simulink model "Hardware_Hidden_Symulink"  (R2022a)
settings: Solver=FixedStepAuto  StartTime=0.0  StopTime=10  FixedStep=1e-3  RelTol=1e-3  EnableMultiTasking=on
undefined symbols (not defined in the file): a, A0, A1, b, c, D0, D1, D10, D11, D12, D13, D2, D3, D5, D6, D8, D9, PTA0, PTA1, PTA2, PTB2, PTB3, PTB9, PTC16, PTC17, PTC2, PTC4, PTD0, PTD1, PTD2, PTD3
libraries: frdmk64flib x19, simulink x1, hdlsllib x1
settings Model: ExtModeTrigDuration=5  Creator=pauls  LastModifiedBy=eddys
settings OptimizationCC: EnhancedBackFolding=on  PassReuseOutputArgsAs=Individual arguments  ZeroExternalMemoryAtStartup=off  ZeroInternalMemoryAtStartup=off  MaxStackSize=64  OptimizeBlockOrder=speed  DifferentSizesBufferReuse=on  OptimizationCustomize=off  EfficientTunableParamExpr=on
settings DebuggingCC: ParameterTunabilityLossMsg=error  UnderSpecifiedDimensionMsg=warning
settings HardwareCC: ProdBitPerPointer=32  ProdBitPerSizeT=32  ProdBitPerPtrDiffT=32  ProdLargestAtomicInteger=Long  ProdLargestAtomicFloat=Double  ProdWordSize=32  ProdHWDeviceType=ARM Compatible->ARM Cortex
settings SFSimCC: MATLABDynamicMemAlloc=off
settings RTWCC: SystemTargetFile=ert.tlc  HardwareBoard=NXP FRDM-K64F  TLCOptions="-aInlineSetEventsForThisBaseRateFcn=TLC_FALSE -aSuppressMultiTaskScheduler=TLC_FALSE  -aRateBasedStepFcn=0"  TemplateMakefile=ert_default_tmf  Toolchain=GNU Tools for ARM Embedded Processors
settings CodeAppCC: ForceParamTrailComments=on  IgnoreCustomStorageClasses=off  OperatorAnnotations=on  SimulinkDataObjDesc=on  SFDataObjDesc=on  InsertBlockDesc=on
settings ERTTargetCC: ExtModeTransport=4  ExtModeMexFile=sendToCommService

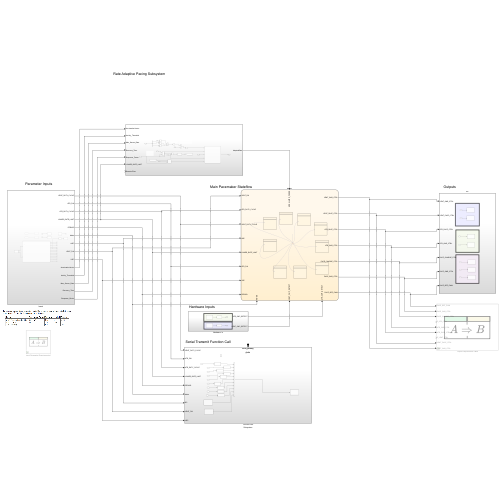
[thumbnail: Simulink's stored preview of the top-level diagram]
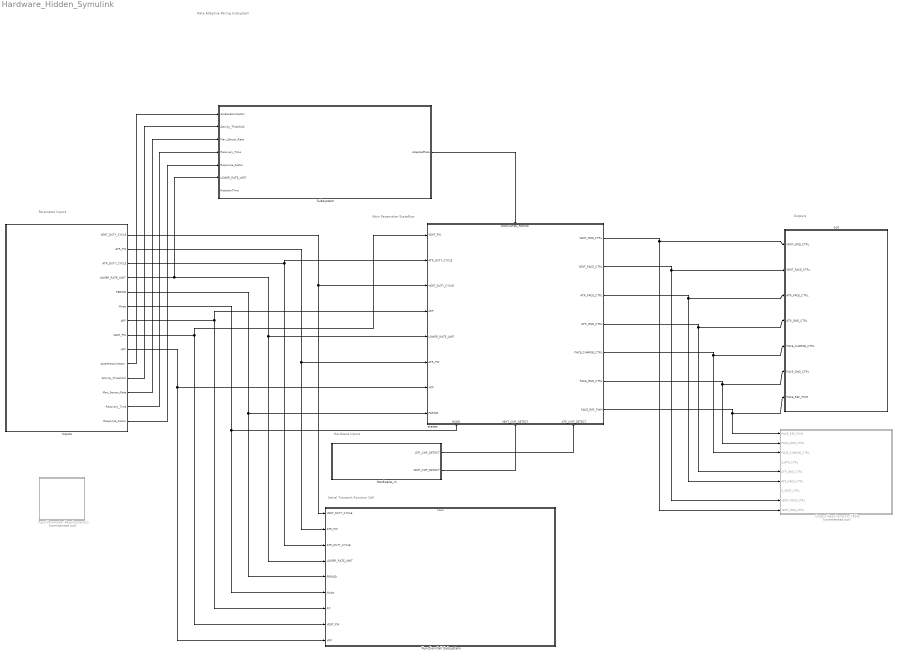
== system Hardware_Hidden_Symulink ==
  note: Rate Adaptive Pacing Subsystem
  note: Serial Transmit Function Call
  note: Main Pacemaker Stateflow
  note: Outputs
  note: Hardware Inputs
  note: Parameter Inputs
  " states  " : Stateflow chart  TreatAsAtomicUnit=on
      settings: PortSchema="{\"entries\":[{\"content\":{\"sides\":[{\"content\":{\"connectorIds\":[\"In4\",\"In6\",\"In5\",\"In10\",\"In11\",\"In7\",\"In9\",\"In8\"]},\"type\":\"ConnectorPlacement.EquallySpacedRectSide\",\"uuid\":\"01118a3a-35ab-415d-a4dc-7a9e5022dc58\"},{\"content\":{\"connectorIds\":[\"Out1\",\"Out2\",\"Out3\",\"Out4\",\"Out5\",\"Out6\",\"Out7\"],\"side\":\"RIGHT\"},\"type\":\"ConnectorPlacement.EquallySpacedRectSide\",\"uuid\":\"d119b6db-c579-45b6-8580-2a3960ab3129\"},{\"content\":{\"connectorIds\":[\"In12\"],\"side\":\"TOP\"},\"type\":\"ConnectorPlacement.EquallySpacedRectSide\",\"uuid\":\"18fa5379-1691-4053-811b-8d647a346445\"},{\"content\":{\"connectorIds\":[\"In1\",\"In3\",\"In2\"],\"side\":\"BOTTOM\"},\"type\":\"ConnectorPlacement.EquallySpacedRectSide\",\"uuid\":\"c19ca9f7-b829-4e11-b03e-3e9d42b35795\"}]},\"type\":\"ConnectorPlacement.EquallySpacedConnector\",\"uuid\":\"6e6fa963-33ea-4c14-97b4-73e5587667a9\"}],\"packageUris\":[\"http://schema.mathworks.com/mf0/Connector/R2020b\"],\"version\":\"1.0\"}"
  Function-Call Subsystem : Subsystem  TreatAsAtomicUnit=on
  Hardware_in : Subsystem
  Input Parameter Requirements1 : Requirements Table  Commented=on  TreatAsAtomicUnit=on
  Inputs : Subsystem
  Output Requirements Table : Requirements Table  Commented=on  TreatAsAtomicUnit=on
  Subsystem : Subsystem
  "out " : Subsystem
  wires:
  Inputs/5(PERIOD) -> Function-Call Subsystem/5(PERIOD), " states  "/8(PERIOD)
  Inputs/4(LOWER_RATE_LIMIT) -> Subsystem/6(LOWER_RATE_LIMIT), Function-Call Subsystem/4(LOWER_RATE_LIMIT), " states  "/11(LOWER_RATE_LIMIT)
  Inputs/1(VENT_DUTY_CYCLE) -> Function-Call Subsystem/1(VENT_DUTY_CYCLE), " states  "/5(VENT_DUTY_CYCLE)
  Inputs/7(ARP) -> Function-Call Subsystem/7(RP), " states  "/10(ARP)
  Inputs/3(ATR_DUTY_CYCLE) -> Function-Call Subsystem/3(ATR_DUTY_CYCLE), " states  "/6(ATR_DUTY_CYCLE)
  Hardware_in/2(VENT_CMP_DETECT) -> " states  "/3(VENT_CMP_DETECT)
  Inputs/2(ATR_PW) -> Function-Call Subsystem/2(ATR_PW), " states  "/7(ATR_PW)
  Hardware_in/1(ATR_CMP_DETECT) -> " states  "/2(ATR_CMP_DETECT)
  Inputs/6(Mode) -> Function-Call Subsystem/6(Mode), " states  "/1(MODE)
  Inputs/8(VENT_PW) -> Function-Call Subsystem/8(VENT_PW), " states  "/4(VENT_PW)
  Inputs/9(VRP) -> Function-Call Subsystem/9(VRP), " states  "/9(VRP)
  " states  "/2(VENT_PACE_CTRL) -> "out "/2(VENT_PACE_CTRL), Output Requirements Table/8(VENT_PACE_CTRL)
  " states  "/7(PACE_REF_PWM) -> Output Requirements Table/1(PACE_REF_PWM), "out "/7(PACE_REF_PWM)
  " states  "/1(VENT_GND_CTRL) -> Output Requirements Table/9(VENT_GND_CTRL), "out "/1(VENT_GND_CTRL)
  " states  "/6(PACE_GND_CTRL) -> Output Requirements Table/2(PACE_GND_CTRL), "out "/6(PACE_GND_CTRL)
  " states  "/3(ATR_PACE_CTRL) -> Output Requirements Table/6(ATR_PACE_CTRL), "out "/3(ATR_PACE_CTRL)
  " states  "/4(ATR_GND_CTRL) -> "out "/4(ATR_GND_CTRL), Output Requirements Table/5(ATR_GND_CTRL)
  " states  "/5(PACE_CHARGE_CTRL) -> Output Requirements Table/3(PACE_CHARGE_CTRL), "out "/5(PACE_CHARGE_CTRL)
  Inputs/10(AccelerationVector) -> Subsystem/1(AccelerationVector)
  Inputs/11(Activity_Threshold) -> Subsystem/2(Activity_Threshold)
  Inputs/12(Max_Sensor_Rate) -> Subsystem/3(Max_Sensor_Rate)
  Inputs/13(Recovery_Time) -> Subsystem/4(Recovery_Time)
  Inputs/14(Response_Factor) -> Subsystem/5(Response_Factor)
  Subsystem/1(AdaptedRate) -> " states  "/12(MODULATED_PERIOD)

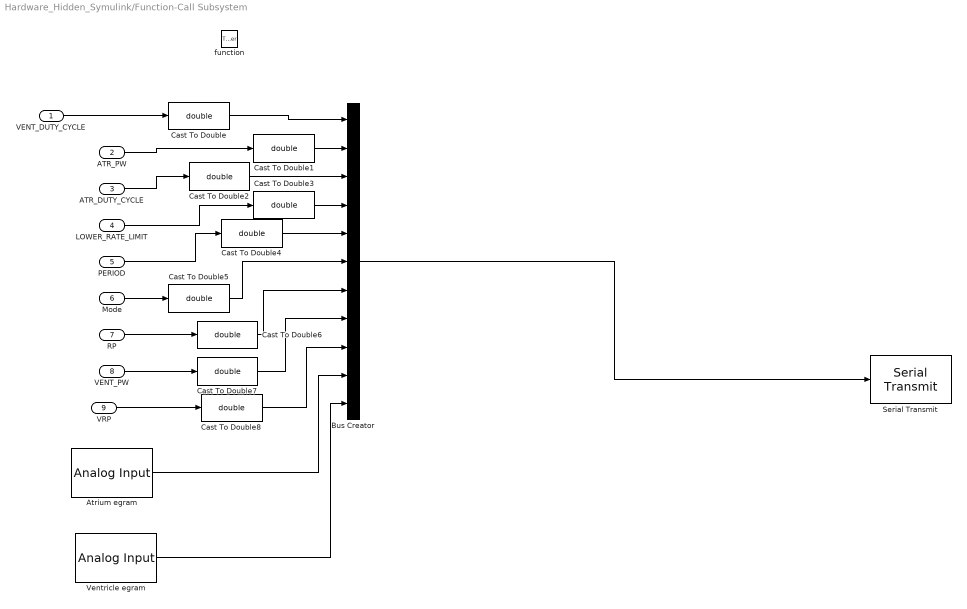
== system Hardware_Hidden_Symulink/Function-Call Subsystem ==
  VENT_DUTY_CYCLE : Inport
  ATR_PW : Inport  Port=2
  ATR_DUTY_CYCLE : Inport  Port=3
  LOWER_RATE_LIMIT : Inport  Port=4
  PERIOD : Inport  Port=5
  Mode : Inport  Port=6
  RP : Inport  Port=7
  VENT_PW : Inport  Port=8
  VRP : Inport  Port=9
  function : TriggerPort  TriggerType=function-call  IsSimulinkFunction=on  FunctionName=send_param  VariantControl=(inherit)
  Atrium egram : frdmk64flib/Analog Input  Whichpin=PTB2 (A0)  SampleTime=-1
  Bus Creator : BusCreator  Inputs=11
  Cast To Double{,1..8} (9 alike) : DataTypeConversion  OutDataTypeStr=double  SaturateOnIntegerOverflow=off  RndMeth=Floor
  Serial Transmit : frdmk64flib/Serial Transmit  SCIModule=0  Baudrate=uint32(9600)  Parity=None  StopBits=1  HardwareFlowControl=None  ByteOrder=LittleEndian  BlockingMode=on  OutputStatus=off
  Ventricle egram : frdmk64flib/Analog Input  Whichpin=PTB3 (A1)  SampleTime=-1
  wires:
  ATR_PW/1 -> Cast To Double1/1
  LOWER_RATE_LIMIT/1 -> Cast To Double3/1
  PERIOD/1 -> Cast To Double4/1
  Mode/1 -> Cast To Double5/1
  RP/1 -> Cast To Double6/1
  VENT_PW/1 -> Cast To Double7/1
  VRP/1 -> Cast To Double8/1
  Bus Creator/1 -> Serial Transmit/1
  Atrium egram/1 -> Bus Creator/10
  Ventricle egram/1 -> Bus Creator/11
  Cast To Double1/1 -> Bus Creator/2
  Cast To Double3/1 -> Bus Creator/4
  Cast To Double4/1 -> Bus Creator/5
  Cast To Double5/1 -> Bus Creator/6
  Cast To Double6/1 -> Bus Creator/7
  Cast To Double7/1 -> Bus Creator/8
  Cast To Double8/1 -> Bus Creator/9
  VENT_DUTY_CYCLE/1 -> Cast To Double/1
  Cast To Double/1 -> Bus Creator/1
  ATR_DUTY_CYCLE/1 -> Cast To Double2/1
  Cast To Double2/1 -> Bus Creator/3

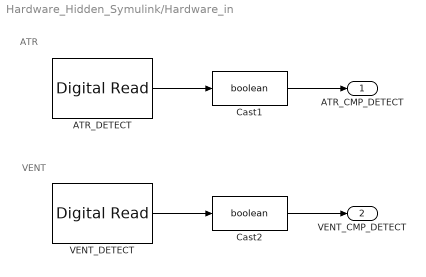
== system Hardware_Hidden_Symulink/Hardware_in ==
  note: VENT
  note: ATR
  ATR_DETECT : frdmk64flib/Digital Read  Whichpin=PTC16 (D0)  SampleTime=-1
  Cast1 : DataTypeConversion  OutDataTypeStr=boolean  SaturateOnIntegerOverflow=off  RndMeth=Floor
  Cast2 : DataTypeConversion  OutDataTypeStr=boolean  SaturateOnIntegerOverflow=off  RndMeth=Floor
  VENT_DETECT : frdmk64flib/Digital Read  Whichpin=PTC17 (D1)  SampleTime=-1
  ATR_CMP_DETECT : Outport
  VENT_CMP_DETECT : Outport  Port=2
  wires:
  Cast1/1 -> ATR_CMP_DETECT/1
  ATR_DETECT/1 -> Cast1/1
  VENT_DETECT/1 -> Cast2/1
  Cast2/1 -> VENT_CMP_DETECT/1

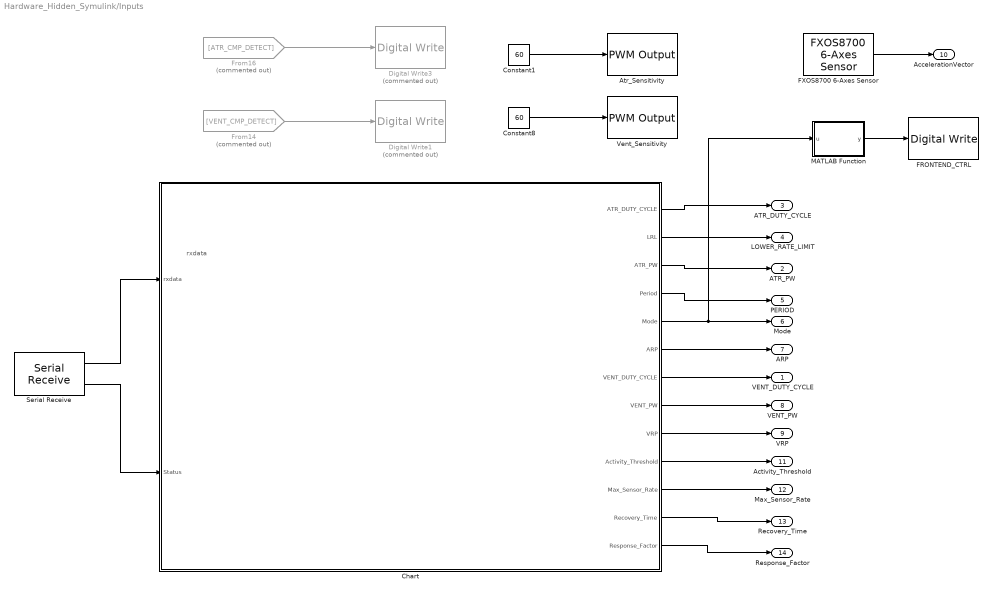
== system Hardware_Hidden_Symulink/Inputs ==
  note: rxdata
  Atr_Sensitivity : frdmk64flib/PWM Output  Whichpin=PTA1 (D3)  InitialFrequency=2000  InitialDutyCycle=0
  Chart : Stateflow chart  TreatAsAtomicUnit=on
      settings: PortSchema="{\"entries\":[{\"content\":{\"sides\":[{\"content\":{\"connectorIds\":[\"In2\",\"In1\"]},\"type\":\"ConnectorPlacement.EquallySpacedRectSide\",\"uuid\":\"d1877822-3205-4f6f-9701-98b371c9c093\"},{\"content\":{\"connectorIds\":[\"Out1\",\"Out2\",\"Out3\",\"Out13\",\"Out4\",\"Out5\",\"Out6\",\"Out7\",\"Out8\",\"Out9\",\"Out10\",\"Out11\",\"Out12\"],\"side\":\"RIGHT\"},\"type\":\"ConnectorPlacement.EquallySpacedRectSide\",\"uuid\":\"d3b9604d-8d2f-41ee-8af9-f72c4df8ba57\"},{\"content\":{\"connectorIds\":[],\"side\":\"TOP\"},\"type\":\"ConnectorPlacement.EquallySpacedRectSide\",\"uuid\":\"4e9204c9-b50b-48f8-942a-bbb1a82b0f42\"}]},\"type\":\"ConnectorPlacement.EquallySpacedConnector\",\"uuid\":\"d64fca82-a3a4-4877-a2ac-6316b03fcfcd\"}],\"packageUris\":[\"http://schema.mathworks.com/mf0/Connector/R2020b\"],\"version\":\"1.0\"}"
  Constant1 : Constant  Value=60
  Constant8 : Constant  Value=60
  Digital Write1 : frdmk64flib/Digital Write  Commented=on  Whichpin=GREEN_LED
  Digital Write3 : frdmk64flib/Digital Write  Commented=on  Whichpin=BLUE_LED
  FRONTEND_CTRL : frdmk64flib/Digital Write  Whichpin=PTD1 (D13)
  FXOS8700 6-Axes Sensor : frdmk64flib/FXOS8700 6-Axes Sensor  Activesensor=Accelerometer only  ODR=800Hz  HybridODR=400Hz  Accelfullrange=-4g to +4g  SampleTime=-1
  From14 : From  Commented=on  GotoTag=VENT_CMP_DETECT
  From16 : From  Commented=on  GotoTag=ATR_CMP_DETECT
  MATLAB Function : MATLAB Function  TreatAsAtomicUnit=on
  Serial Receive : frdmk64flib/Serial Receive  SCIModule=0  Baudrate=uint32(9600)  Parity=None  StopBits=1  HardwareFlowControl=None  ByteOrder=LittleEndian  DataType=uint8  DataLength=19  BlockingMode=off  OutputStatus=on  SampleTime=0.1
  Vent_Sensitivity : frdmk64flib/PWM Output  Whichpin=PTC2 (D6)  InitialFrequency=2000  InitialDutyCycle=0
  VENT_DUTY_CYCLE : Outport
  ATR_PW : Outport  Port=2
  ATR_DUTY_CYCLE : Outport  Port=3
  LOWER_RATE_LIMIT : Outport  Port=4
  PERIOD : Outport  Port=5
  Mode : Outport  Port=6
  ARP : Outport  Port=7
  VENT_PW : Outport  Port=8
  VRP : Outport  Port=9
  AccelerationVector : Outport  Port=10
  Activity_Threshold : Outport  Port=11
  Max_Sensor_Rate : Outport  Port=12
  Recovery_Time : Outport  Port=13
  Response_Factor : Outport  Port=14
  wires:
  From14/1 -> Digital Write1/1
  Constant8/1 -> Vent_Sensitivity/1
  Constant1/1 -> Atr_Sensitivity/1
  From16/1 -> Digital Write3/1
  Chart/1(ATR_DUTY_CYCLE) -> ATR_DUTY_CYCLE/1
  Chart/2(LRL) -> LOWER_RATE_LIMIT/1
  Chart/3(ATR_PW) -> ATR_PW/1
  Chart/6(VENT_DUTY_CYCLE) -> VENT_DUTY_CYCLE/1
  Serial Receive/2 -> Chart/1(Status)
  Serial Receive/1 -> Chart/2(rxdata)
  Chart/4(Mode) -> MATLAB Function/1(u), Mode/1
  Chart/5(ARP) -> ARP/1
  Chart/7(VENT_PW) -> VENT_PW/1
  Chart/8(VRP) -> VRP/1
  MATLAB Function/1(y) -> FRONTEND_CTRL/1
  FXOS8700 6-Axes Sensor/1 -> AccelerationVector/1
  Chart/9(Activity_Threshold) -> Activity_Threshold/1
  Chart/10(Max_Sensor_Rate) -> Max_Sensor_Rate/1
  Chart/11(Recovery_Time) -> Recovery_Time/1
  Chart/12(Response_Factor) -> Response_Factor/1
  Chart/13(Period) -> PERIOD/1

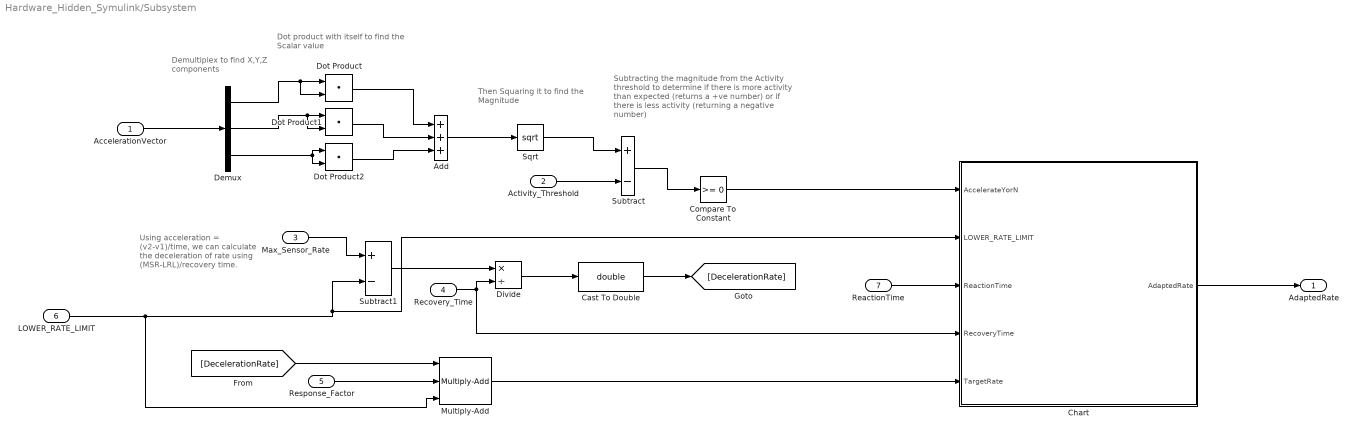
== system Hardware_Hidden_Symulink/Subsystem ==
  note: Demultiplex to find
      | X,Y,Z components
  note: Using acceleration = (v2-v1)/time, we can calculate the deceleration of rate using
      | (MSR-LRL)/recovery time.
  note: Subtracting the magnitude from the Activity threshold to determine if there is more activity than expected (returns a +ve number) or if there is less activity (returning a negative number)
  note: Dot product with itself to find the
      | Scalar value
  note: Then Squaring it to find the Magnitude
  AccelerationVector : Inport
  Activity_Threshold : Inport  Port=2
  Max_Sensor_Rate : Inport  Port=3
  Recovery_Time : Inport  Port=4
  Response_Factor : Inport  Port=5
  LOWER_RATE_LIMIT : Inport  Port=6
  ReactionTime : Inport  Port=7
  Add : Sum  Inputs=+++
  Cast To Double : DataTypeConversion  OutDataTypeStr=double  SaturateOnIntegerOverflow=off  RndMeth=Floor
  Chart : Stateflow chart  TreatAsAtomicUnit=on
      settings: PortSchema="{\"entries\":[{\"content\":{\"sides\":[{\"content\":{\"connectorIds\":[\"In2\",\"In1\",\"In3\",\"In4\",\"In5\"]},\"type\":\"ConnectorPlacement.EquallySpacedRectSide\",\"uuid\":\"6eaaa5c3-a67e-4334-8771-4d714dd3c2aa\"},{\"content\":{\"connectorIds\":[\"Out1\"],\"side\":\"RIGHT\"},\"type\":\"ConnectorPlacement.EquallySpacedRectSide\",\"uuid\":\"be5e1652-7b89-433f-97fe-a51584ee4ad6\"},{\"content\":{\"connectorIds\":[],\"side\":\"TOP\"},\"type\":\"ConnectorPlacement.EquallySpacedRectSide\",\"uuid\":\"88923a53-eca7-4a95-abe6-229d007878e0\"}]},\"type\":\"ConnectorPlacement.EquallySpacedConnector\",\"uuid\":\"0db105c6-87da-444f-9a1d-26abcd68563f\"}],\"packageUris\":[\"http://schema.mathworks.com/mf0/Connector/R2020b\"],\"version\":\"1.0\"}"
  Compare To Constant : simulink/Logic and Bit Operations/Compare To Constant  relop=>=  const=0  OutDataTypeStr=boolean
  Demux : Demux  Outputs=3
  Divide : Product  Inputs=*/
  Dot Product : DotProduct  OutDataTypeStr=Inherit: Inherit via internal rule
  Dot Product1 : DotProduct  OutDataTypeStr=Inherit: Inherit via internal rule
  Dot Product2 : DotProduct  OutDataTypeStr=Inherit: Inherit via internal rule
  Multiply-Add : hdlsllib/HDL Operations/Multiply-Add  Function=c+(a.*b)  datatype=Inherit: Inherit via internal rule  DoSatur=off  FMA=off
      settings: SourceProductBaseCode=SL
  Sqrt : Sqrt
  Subtract : Sum  Inputs=+-
  Subtract1 : Sum  Inputs=+-
  AdaptedRate : Outport
  wires:
  AccelerationVector/1 -> Demux/1
  Dot Product/1 -> Add/1
  Sqrt/1 -> Subtract/1
  Activity_Threshold/1 -> Subtract/2
  Subtract/1 -> Compare To Constant/1
  LOWER_RATE_LIMIT/1 -> Multiply-Add/3, Subtract1/2, Chart/1(LOWER_RATE_LIMIT)
  Max_Sensor_Rate/1 -> Subtract1/1
  Subtract1/1 -> Divide/1
  Recovery_Time/1 -> Chart/4(RecoveryTime), Divide/2
  Divide/1 -> Cast To Double/1
  Response_Factor/1 -> Multiply-Add/2
  Add/1 -> Sqrt/1
  Demux/1 -> Dot Product/2, Dot Product/1
  Demux/3 -> Dot Product2/2, Dot Product2/1
  Demux/2 -> Dot Product1/2, Dot Product1/1
  Dot Product1/1 -> Add/2
  Dot Product2/1 -> Add/3
  Cast To Double/1 -> [DecelerationRate]
  [DecelerationRate] -> Multiply-Add/1
  Compare To Constant/1 -> Chart/2(AccelerateYorN)
  ReactionTime/1 -> Chart/3(ReactionTime)
  Multiply-Add/1 -> Chart/5(TargetRate)
  Chart/1(AdaptedRate) -> AdaptedRate/1

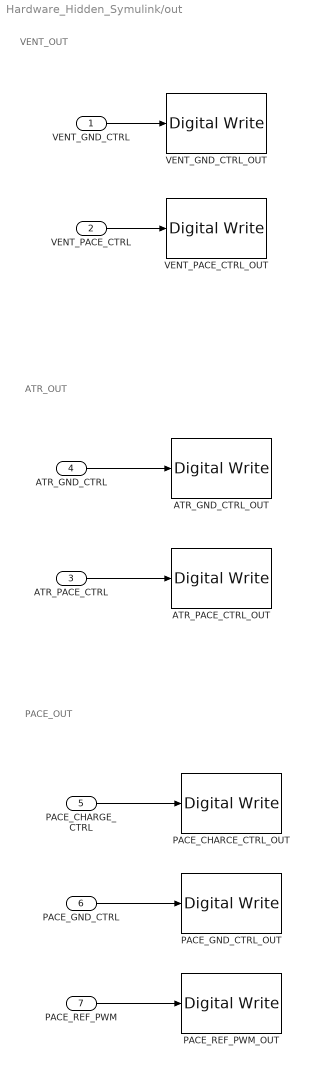
== system Hardware_Hidden_Symulink/out  ==
  note: PACE_OUT
  note: ATR_OUT
  note: VENT_OUT
  VENT_GND_CTRL : Inport
  VENT_PACE_CTRL : Inport  Port=2
  ATR_PACE_CTRL : Inport  Port=3
  ATR_GND_CTRL : Inport  Port=4
  PACE_CHARGE_CTRL : Inport  Port=5
  PACE_GND_CTRL : Inport  Port=6
  PACE_REF_PWM : Inport  Port=7
  ATR_GND_CTRL_OUT : frdmk64flib/Digital Write  Whichpin=PTD2 (D11)
  ATR_PACE_CTRL_OUT : frdmk64flib/Digital Write  Whichpin=PTA0 (D8)
  PACE_CHARCE_CTRL_OUT : frdmk64flib/Digital Write  Whichpin=PTB9 (D2)
  PACE_GND_CTRL_OUT : frdmk64flib/Digital Write  Whichpin=PTD0 (D10)
  PACE_REF_PWM_OUT : frdmk64flib/Digital Write  Whichpin=PTA2 (D5)
  VENT_GND_CTRL_OUT : frdmk64flib/Digital Write  Whichpin=PTD3 (D12)
  VENT_PACE_CTRL_OUT : frdmk64flib/Digital Write  Whichpin=PTC4 (D9)
  wires:
  VENT_GND_CTRL/1 -> VENT_GND_CTRL_OUT/1
  VENT_PACE_CTRL/1 -> VENT_PACE_CTRL_OUT/1
  ATR_GND_CTRL/1 -> ATR_GND_CTRL_OUT/1
  ATR_PACE_CTRL/1 -> ATR_PACE_CTRL_OUT/1
  PACE_CHARGE_CTRL/1 -> PACE_CHARCE_CTRL_OUT/1
  PACE_REF_PWM/1 -> PACE_REF_PWM_OUT/1
  PACE_GND_CTRL/1 -> PACE_GND_CTRL_OUT/1

== stateflow chart Hardware_Hidden_Symulink/Inputs/Chart ==
  state Set_Param
    entry:
    %These will be changed to rxdata(#) and typecasted
    ATR_DUTY_CYCLE = rxdata(3);
    ATR_PW = rxdata(4);
    Mode = rxdata(5);
    VENT_DUTY_CYCLE =rxdata(6);
    VENT_PW = rxdata(7);
    ARP = rxdata(8);
    VRP = rxdata(9);
    LRL = rxdata(10);
    Period = 60000/LRL;
    %Rate Adaptive Pacing Parameters
    Activity_Threshold =rxdata(11);
    Response_Factor =rxdata(12);
    Recovery_Time = rxdata(13);
    Max_Sensor_Rate =rxdata(14);
  state Initial
    entry:
    ATR_DUTY_CYCLE = 1;
    ATR_PW = 1;
    Mode =1;
    VENT_DUTY_CYCLE =1;
    VENT_PW = 1;
    ARP =1;
    VRP = 1;
    LRL = 1;
    Period = 60000/LRL;
    Activity_Threshold =1;
    Response_Factor =1;
    Recovery_Time = 1;
    Max_Sensor_Rate =1;
  state StandBy
    %Waiting for communication from
    %the DCM
  state Echo_Param
    entry:
    send_param();
  Set_Param -> StandBy
  (default) -> Initial
  (junction 14) -> Set_Param [order 1] : [rxdata(2)==hex2dec('55')]
  (junction 12) -> StandBy [order 2]
  StandBy -> (junction 12) : [Status == 0]
  (junction 12) -> (junction 14) [order 1] : [rxdata(1) == hex2dec('16')]
  Initial -> StandBy
  (junction 14) -> Echo_Param [order 2] : [rxdata(2) == hex2dec('22')]
  Echo_Param -> StandBy
  data: Status input; rxdata input; ATR_DUTY_CYCLE output; LRL output; ATR_PW output; Mode output; ARP output; VENT_DUTY_CYCLE output; VENT_PW output; VRP output; Activity_Threshold output; Max_Sensor_Rate output; Recovery_Time output; Response_Factor output; Period output

== matlab function Hardware_Hidden_Symulink/Inputs/MATLAB Function ==
  data: u input; y output
function y = fcn(u)

if (u == 3||u == 4||u == 7||u == 8)
    y=1;
else
    y=0;
end

== stateflow chart Hardware_Hidden_Symulink/ states   ==
  state Default [group]
    state CharingC23
      during:
      %Begin Charging C22 Capacitor
      VENT_PACE_CTRL = LOW;
      PACE_REF_PWM = VENT_DUTY_CYCLE;
      PACE_CHARGE_CTRL = HIGH;
      %Begin Discharging C21 Blocking Capacitor
      PACE_GND_CTRL = HIGH;
      VENT_PACE_CTRL = LOW;
      VENT_GND_CTRL = HIGH;
    state Discharge
      during:
      %Discharge C22 into Ventricle (Vent Pacing)
      %Begin Charging Blocking Capacitor
      PACE_CHARGE_CTRL = LOW;
      PACE_GND_CTRL = HIGH;
      VENT_GND_CTRL = LOW;
      VENT_PACE_CTRL  = HIGH;
    Default.CharingC23 -> Default.Discharge : after(PERIOD-VENT_PW, msec)
    Default.Discharge -> Default.CharingC23 : after(VENT_PW, msec)
  state AOO [group]
    state CharingC22
      %Capacitor charing state
      ATR_PACE_CTRL = LOW
      PACE_REF_PWM = ATR_DUTY_CYCLE
      PACE_CHARGE_CTRL = HIGH
      %Discharge capacitor
      PACE_GND_CTRL = HIGH
      ATR_PACE_CTRL = LOW
      ATR_GND_CTRL = HIGH
    state AVPacing
      %step 2
      PACE_CHARGE_CTRL = LOW
      PACE_GND_CTRL = HIGH
      ATR_PACE_CTRL = HIGH
      ATR_GND_CTRL = LOW
    AOO.CharingC22 -> AOO.AVPacing : after(PERIOD-ATR_PW, msec)
    AOO.AVPacing -> AOO.CharingC22 : after(ATR_PW, msec)
  state VVIR [group]
    state DISCHARGING
      during:
      %Step 1:
      %Discharge C22 into Ventricle (Vent Pacing)
      %Begin Charging Blocking Capacitor
      PACE_CHARGE_CTRL = LOW
      PACE_GND_CTRL = HIGH
      VENT_GND_CTRL = LOW
      VENT_PACE_CTRL  = HIGH
    state CHARGING
      during:
      %Begin Charging C22 Capacitor
      VENT_PACE_CTRL = LOW;
      PACE_REF_PWM = VENT_DUTY_CYCLE;
      PACE_CHARGE_CTRL = HIGH;
      %Begin Discharging C21 Blocking Capacitor
      PACE_GND_CTRL = HIGH;
      VENT_PACE_CTRL = LOW;
      VENT_GND_CTRL = HIGH;
    state PROXY
      during:
      PACE_GND_CTRL = HIGH;
      VENT_PACE_CTRL = LOW;
      VENT_GND_CTRL = HIGH;
    CHARGING -> VVIR.DISCHARGING : after(MODULATED_PERIOD-VENT_PW-VRP, msec)
    VVIR.DISCHARGING -> (junction 195) [order 2] : after(LOWER_RATE_LIMIT,msec)
    (junction 195) -> PROXY : [VENT_CMP_DETECT==HIGH]
    VVIR.DISCHARGING -> PROXY [order 1] : after(VENT_PW, msec)
    PROXY -> CHARGING : after(VRP, msec)
  state VOO [group]
    state CharingC23
      during:
      %Begin Charging C22 Capacitor
      VENT_PACE_CTRL = LOW;
      PACE_REF_PWM = VENT_DUTY_CYCLE;
      PACE_CHARGE_CTRL = HIGH;
      %Begin Discharging C21 Blocking Capacitor
      PACE_GND_CTRL = HIGH;
      VENT_PACE_CTRL = LOW;
      VENT_GND_CTRL = HIGH;
    state Discharge
      during:
      %Discharge C22 into Ventricle (Vent Pacing)
      %Begin Charging Blocking Capacitor
      PACE_CHARGE_CTRL = LOW;
      PACE_GND_CTRL = HIGH;
      VENT_GND_CTRL = LOW;
      VENT_PACE_CTRL  = HIGH;
    VOO.CharingC23 -> VOO.Discharge : after(PERIOD-VENT_PW, msec)
    VOO.Discharge -> VOO.CharingC23 : after(VENT_PW, msec)
  state AAIR [group]
    state DISCHARGING
      during:
      %Discharge C22 into Atrium (Atrial Pacing)
      %Begin Charging Blocking Capacitor
      PACE_CHARGE_CTRL = LOW
      PACE_GND_CTRL = HIGH
      ATR_PACE_CTRL = HIGH
      ATR_GND_CTRL = LOW
    state CharingC23
      during:
      %Begin Charging C22 Capacitor
      ATR_PACE_CTRL = LOW
      PACE_REF_PWM = ATR_DUTY_CYCLE
      PACE_CHARGE_CTRL = HIGH
      %Begin Discharging C21 Blocking Capacitor
      PACE_GND_CTRL = HIGH
      ATR_PACE_CTRL = LOW
      ATR_GND_CTRL = HIGH
    state Proxy
      during:
      PACE_GND_CTRL = HIGH
      ATR_PACE_CTRL = LOW
      ATR_GND_CTRL = HIGH
    AAIR.CharingC23 -> AAIR.DISCHARGING : after(MODULATED_PERIOD-ATR_PW-ARP, msec)
    AAIR.DISCHARGING -> (junction 178) [order 2] : after(LOWER_RATE_LIMIT,msec)
    (junction 178) -> Proxy : [ATR_CMP_DETECT==HIGH]
    AAIR.DISCHARGING -> Proxy [order 1] : after(ATR_PW, msec)
    Proxy -> AAIR.CharingC23 : after(ARP, msec)
  state VVI [group]
    state Discharge
      during:
      %Discharge C22 into Ventricle (Vent Pacing)
      %Begin Charging Blocking Capacitor
      PACE_CHARGE_CTRL = LOW
      PACE_GND_CTRL = HIGH
      VENT_GND_CTRL = LOW
      VENT_PACE_CTRL  = HIGH
    state CharingC23
      during:
      %Begin Charging C22 Capacitor
      VENT_PACE_CTRL = LOW;
      PACE_REF_PWM = VENT_DUTY_CYCLE;
      PACE_CHARGE_CTRL = HIGH;
      %Begin Discharging C21 Blocking Capacitor
      PACE_GND_CTRL = HIGH;
      VENT_PACE_CTRL = LOW;
      VENT_GND_CTRL = HIGH;
    state Inhibit
      PACE_GND_CTRL = HIGH
      VENT_PACE_CTRL = LOW
      VENT_GND_CTRL = HIGH
    VVI.CharingC23 -> VVI.Discharge [order 1] : after(PERIOD-VENT_PW, msec)[VENT_CMP_DETECT == LOW]
    VVI.CharingC23 -> VVI.Inhibit [order 2] : after(LOWER_RATE_LIMIT, msec)[VENT_CMP_DETECT == HIGH]
    VVI.Inhibit -> VVI.CharingC23 : after(VRP,msec)
    VVI.Discharge -> VVI.Inhibit : after(VENT_PW, msec)
  state AAI [group]
    state AVPacing
      %step 2
      PACE_CHARGE_CTRL = LOW
      PACE_GND_CTRL = HIGH
      ATR_PACE_CTRL = HIGH
      ATR_GND_CTRL = LOW
    state CharingC22
      %Capacitor charing state
      ATR_PACE_CTRL = LOW
      PACE_REF_PWM = ATR_DUTY_CYCLE
      PACE_CHARGE_CTRL = HIGH
      %Discharge capacitor
      PACE_GND_CTRL = HIGH
      ATR_PACE_CTRL = LOW
      ATR_GND_CTRL = HIGH
    state Inhibit
      %Through Trial and error found that discharging
      %again will fix the pacing during AAI
      PACE_GND_CTRL = HIGH
      ATR_PACE_CTRL = LOW
      ATR_GND_CTRL = LOW
    AAI.CharingC22 -> AAI.AVPacing [order 2] : after(PERIOD-ATR_PW, msec)
    AAI.CharingC22 -> AAI.Inhibit [order 1] : after(LOWER_RATE_LIMIT,msec)[ATR_CMP_DETECT == HIGH]
    AAI.AVPacing -> AAI.Inhibit : after(ATR_PW, msec)
    AAI.Inhibit -> AAI.CharingC22 : after(ARP,msec)
  state AOOR [group]
    state CharingC23
      during:
      %Begin Charging C22 Capacitor
      ATR_PACE_CTRL = LOW
      PACE_REF_PWM = ATR_DUTY_CYCLE
      PACE_CHARGE_CTRL = HIGH
      %Begin Discharging C21 Blocking Capacitor
      PACE_GND_CTRL = HIGH
      ATR_PACE_CTRL = LOW
      ATR_GND_CTRL = HIGH
    state AVPacing1
      during:
      %Discharge C22 into Ventricle (Vent Pacing)
      %Begin Charging Blocking Capacitor
      PACE_CHARGE_CTRL = LOW
      PACE_GND_CTRL = HIGH
      ATR_GND_CTRL = LOW
      ATR_PACE_CTRL  = HIGH
    AOOR.CharingC23 -> AOOR.AVPacing1 : after(PERIOD-ATR_PW, msec)
    AOOR.AVPacing1 -> AOOR.CharingC23 : after(ATR_PW, msec)
  state VOOR [group]
    state CharingC23
      during:
      %Begin Charging C22 Capacitor
      VENT_PACE_CTRL = LOW
      PACE_REF_PWM = VENT_DUTY_CYCLE
      PACE_CHARGE_CTRL = HIGH
      %Begin Discharging C21 Blocking Capacitor
      PACE_GND_CTRL = HIGH
      VENT_PACE_CTRL = LOW
      VENT_GND_CTRL = HIGH
    state AVPacing1
      during:
      %Discharge C22 into Ventricle (Vent Pacing)
      %Begin Charging Blocking Capacitor
      PACE_CHARGE_CTRL = LOW
      PACE_GND_CTRL = HIGH
      VENT_GND_CTRL = LOW
      VENT_PACE_CTRL  = HIGH
    VOOR.CharingC23 -> VOOR.AVPacing1 : after(PERIOD-ATR_PW, msec)
    VOOR.AVPacing1 -> VOOR.CharingC23 : after(ATR_PW, msec)
  (junction 211) -> CHARGING [order 8] : [MODE==8]
  (junction 211) -> Default.CharingC23 [order 9]
  (default) -> (junction 211)
  (junction 211) -> VOOR.CharingC23 [order 6] : [MODE == 6]
  (junction 211) -> AAIR.CharingC23 [order 7] : [MODE == 7]
  (junction 211) -> AOOR.CharingC23 [order 5] : [MODE ==5]
  (junction 211) -> VVI.CharingC23 [order 3] : [MODE ==3]
  (junction 211) -> AAI.CharingC22 [order 4] : [MODE == 4]
  (junction 211) -> AOO.CharingC22 [order 1] : [MODE ==1]
  (junction 211) -> VOO.CharingC23 [order 2] : [MODE ==2]
  data: MODE input; ATR_CMP_DETECT input; VENT_CMP_DETECT input; VENT_GND_CTRL output; VENT_PACE_CTRL output; ATR_PACE_CTRL output; VENT_PW input; VENT_DUTY_CYCLE input; HIGH local =true; LOW local =false; ATR_GND_CTRL output; PACE_CHARGE_CTRL output; PACE_GND_CTRL output; PACE_REF_PWM output; ATR_DUTY_CYCLE input; ATR_PW input; PERIOD input; VRP input; ARP input; LOWER_RATE_LIMIT input; MODULATED_PERIOD input

== stateflow chart Hardware_Hidden_Symulink/Output Requirements Table ==
  (default) -> (junction 1073741860)
  (junction 1073741860) -> (junction 1073741861) : {
      | % SF_REQ_REV_07
      | }
  (junction 1073741861) -> (junction 1073741863) : {
      | % HEADER_ASSIGNMENTS
      |
      | }
  (junction 1073741863) -> (junction 1073741865) : {
      | % START_A_4
      | }
  (junction 1073741865) -> (junction 1073741867) : {
      | }
  (junction 1073741867) -> (junction 1073741869)
  (junction 1073741869) -> (junction 1073741871) : {
      | }
  (junction 1073741871) -> (junction 1073741873) : {
      | % END_A_4
      | }
  (junction 1073741873) -> (junction 1073741898) : {
      | % START_R_1
      | }
  (junction 1073741898) -> (junction 1073741900) : {
      | }
  (junction 1073741900) -> (junction 1073741902) : {
      |
      |
      | }
  (junction 1073741902) -> (junction 1073741904) : {
      | }
  (junction 1073741904) -> (junction 1073741906) : {
      | % END_R_1
      | }
  data: PACE_REF_PWM input; PACE_GND_CTRL input; PACE_CHARGE_CTRL input; Z_ATR_CTRL input; ATR_GND_CTRL input; ATR_PACE_CTRL input; Z_VENT_CTRL input; VENT_PACE_CTRL input; VENT_GND_CTRL input

== stateflow chart Hardware_Hidden_Symulink/Input Parameter Requirements1 ==
  (default) -> (junction 1073741930)
  (junction 1073741930) -> (junction 1073741931) : {
      | % SF_REQ_REV_07
      | }
  (junction 1073741931) -> (junction 1073741933) : {
      | % HEADER_ASSIGNMENTS
      |
      | }
  (junction 1073741933) -> (junction 1073741935) : {
      | % START_A_4
      | }
  (junction 1073741935) -> (junction 1073741937) : {
      | }
  (junction 1073741937) -> (junction 1073741939)
  (junction 1073741939) -> (junction 1073741941) : {
      | }
  (junction 1073741941) -> (junction 1073741943) : {
      | % END_A_4
      | }
  (junction 1073741943) -> (junction 1073741945) : {
      | % START_R_1
      | }
  (junction 1073741945) -> (junction 1073741947) : {
      | }
  (junction 1073741947) -> (junction 1073741949)
  (junction 1073741949) -> (junction 1073741951) [order 1] : [(((p_aPaceAmp) == (0 || [0.112, 5.6]))) && (((p_vPaceAmp) == (0 || [0.112, 5.6]))) && (((p_aPaceWidth) >= (1) && (p_aPaceWidth) <= (31))) && (((p_vPaceWidth) >= (1) && (p_vPaceWidth) <= (31))) && (((p_aSensitivity) >= (0) && (p_aSensitivity) <= (5))) && (((p_vSensitivity) >= (0) && (p_vSensitivity) <= (5))) && ([150,500] && p_aPaceWidth < (p_ARP)< p_lowrateInterval) && ([150,500] && p_vPaceWidth < (p_VRP) < p_lowrateInterval) && (((p_lowrateInterval ) >= (343) && (p_lowrateInterval ) <= (2000))) && (((p_pacingMode ) == (1)) || ((p_pacingMode ) == (2)) || ((p_pacingMode ) == (3)) || ((p_pacingMode ) == (4)) || ((p_pacingMode ) == (5)))]
  (junction 1073741949) -> (junction 1073741957) [order 2]
  (junction 1073741951) -> (junction 1073741953) : {
      | Pass
      |
      | }
  (junction 1073741953) -> (junction 1073741955) : {
      | }
  (junction 1073741955) -> (junction 1073741957)
  (junction 1073741957) -> (junction 1073741959)
  (junction 1073741959) -> (junction 1073741961) : {
      | % END_R_1
      | }

== stateflow chart Hardware_Hidden_Symulink/Subsystem/Chart ==
  state S2FAIL1
    entry:
    AdaptedRate = AdaptedRate - step_down;
  state S4
    entry:
    AdaptedRate = AdaptedRate + step_up;
  state S3
    entry:
    AdaptedRate = TargetRate;
  state Start1
    entry:
    AdaptedRate = LOWER_RATE_LIMIT;
  state S_FAILSAFE1
    entry:
    AdaptedRate = AdaptedRate - step_up;
  S_FAILSAFE1 -> S2FAIL1 [order 2] : [ after(1000,msec)]
  S2FAIL1 -> Start1 [order 1] : [AdaptedRate <= LOWER_RATE_LIMIT]
  S2FAIL1 -> S2FAIL1 [order 2] : after(1000, msec)[AdaptedRate >= LOWER_RATE_LIMIT]
  S2FAIL1 -> S4 [order 3] : [AccelerateYorN == 1]
  S3 -> S2FAIL1 [order 2] : [AccelerateYorN == 0]
  (default) -> Start1 : {step_up = ceil((TargetRate - LOWER_RATE_LIMIT) / ReactionTime),
      | step_down = ceil((TargetRate - LOWER_RATE_LIMIT)  / RecoveryTime)}
  S4 -> S4 [order 1] : after(1000,msec)[AdaptedRate <= TargetRate]
  S4 -> S3 [order 3] : [AdaptedRate >= TargetRate]
  Start1 -> S4 [order 1] : [AccelerateYorN == 1]
  Start1 -> Start1 [order 2] : [AccelerateYorN == 0]
  S3 -> S3 [order 1] : [AccelerateYorN == 1]
  S4 -> S_FAILSAFE1 [order 2] : [AccelerateYorN == 0]
  S_FAILSAFE1 -> S4 [order 1] : [AccelerateYorN == 1]
  data: step_down local; step_up local; LOWER_RATE_LIMIT input; AccelerateYorN input; ReactionTime input; RecoveryTime input; AdaptedRate output; TargetRate input
